simulink model "sensors"  (R2026a)
settings: Solver=VariableStepAuto
undefined symbols (not defined in the file): fractalcoef
libraries: mspsensorlib x1
settings Model: Creator=arroy  LastModifiedBy=Owner

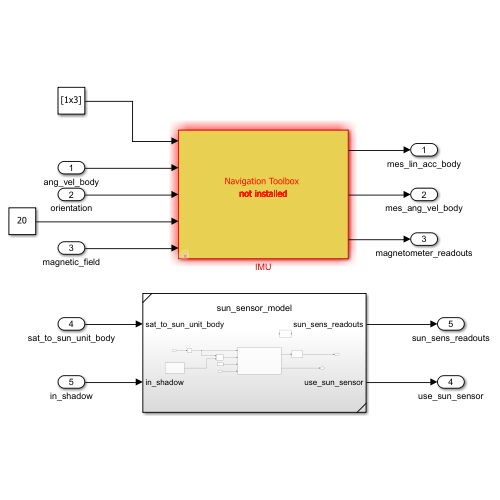
[thumbnail: Simulink's stored preview of the top-level diagram]
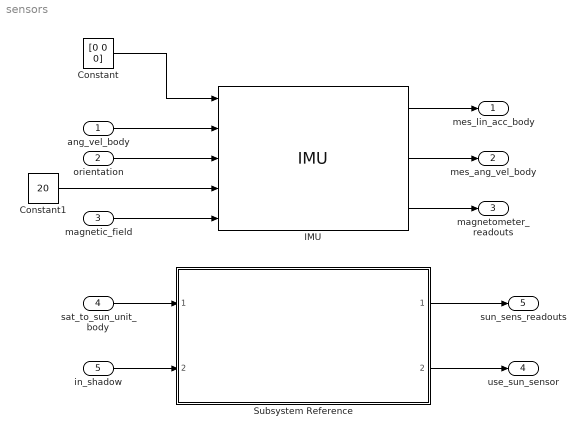
== system sensors ==
  ang_vel_body : Inport
  orientation : Inport  Port=2
  magnetic_field : Inport  Port=3
  sat_to_sun_unit_body : Inport  Port=4
  in_shadow : Inport  Port=5
  Constant : Constant  Value=[0 0 0]
  Constant1 : Constant  Value=20
  IMU : mspsensorlib/IMU  DispRefFrame=NED  TemperaturePort=on  Temperature=25  MagneticFieldPort=on  MagneticFieldNED=[ 27.5550, -2.4169, -16.0849 ]  MagneticFieldENU=[ -2.4169, 27.5550, 16.0849 ]  SeedDouble=67  SimulateUsing=Interpreted execution  AccelParamsMeasurementRange=Inf  AccelParamsResolution=0  AccelParamsConstantBias=[ 0, 0, 0 ]  AccelParamsAxesMisalignment=[ 100, 0, 0; 0, 100, 0; 0, 0, 100 ]  AccelParamsNoiseDensity=[ 0, 0, 0 ]  AccelParamsBiasInstability=[ 0, 0, 0 ]  AccelParamsBiasInstabilityNumerator=fractalcoef().Numerator  AccelParamsBiasInstabilityDenominator=fractalcoef().Denominator  AccelParamsRandomWalk=[ 0, 0, 0 ]  AccelParamsNoiseType=double-sided  AccelParamsTemperatureBias=[ 0, 0, 0 ]  AccelParamsTemperatureScaleFactor=[ 0, 0, 0 ]  GyroParamsMeasurementRange=Inf  GyroParamsResolution=0  GyroParamsConstantBias=[ 0, 0, 0 ]  GyroParamsAxesMisalignment=[ 100, 0, 0; 0, 100, 0; 0, 0, 100 ]  GyroParamsAccelerationBias=[ 0, 0, 0 ]  GyroParamsNoiseDensity=[ 0, 0, 0 ]  GyroParamsBiasInstability=[ 0, 0, 0 ]  GyroParamsBiasInstabilityNumerator=fractalcoef().Numerator  GyroParamsBiasInstabilityDenominator=fractalcoef().Denominator  GyroParamsRandomWalk=[ 0, 0, 0 ]  GyroParamsNoiseType=double-sided  GyroParamsTemperatureBias=[ 0, 0, 0 ]  GyroParamsTemperatureScaleFactor=[ 0, 0, 0 ]  MagParamsMeasurementRange=Inf  MagParamsResolution=0  MagParamsConstantBias=[ 0, 0, 0 ]  MagParamsAxesMisalignment=[ 100, 0, 0; 0, 100, 0; 0, 0, 100 ]  MagParamsNoiseDensity=[ 0, 0, 0 ]  MagParamsBiasInstability=[ 0, 0, 0 ]  MagParamsBiasInstabilityNumerator=fractalcoef().Numerator  MagParamsBiasInstabilityDenominator=fractalcoef().Denominator  MagParamsRandomWalk=[ 0, 0, 0 ]  MagParamsNoiseType=double-sided  MagParamsTemperatureBias=[ 0, 0, 0 ]  MagParamsTemperatureScaleFactor=[ 0, 0, 0 ]
  Subsystem Reference : Subsystem  ReferencedSubsystem=sun_sensor_model
  mes_lin_acc_body : Outport
  mes_ang_vel_body : Outport  Port=2
  magnetometer_readouts : Outport  Port=3
  use_sun_sensor : Outport  Port=4
  sun_sens_readouts : Outport  Port=5
  wires:
  Constant/1 -> IMU/1
  ang_vel_body/1 -> IMU/2
  orientation/1 -> IMU/3
  Constant1/1 -> IMU/4
  sat_to_sun_unit_body/1 -> Subsystem Reference/1
  magnetic_field/1 -> IMU/5
  in_shadow/1 -> Subsystem Reference/2
  IMU/1 -> mes_lin_acc_body/1
  IMU/2 -> mes_ang_vel_body/1
  IMU/3 -> magnetometer_readouts/1
  Subsystem Reference/2 -> use_sun_sensor/1
  Subsystem Reference/1 -> sun_sens_readouts/1
